simulink model "model_user_tracking"  (R2023a)
settings: Solver=VariableStepAuto  StartTime=0.0  StopTime=10.0  RelTol=1e-3
InitFcn:
  | f = 20%Hz
  | Robot_Start = [0,0];
  | User_Start = [-1,-1];
  | User_Speed = 1;
  | D_Accuracy = 0.25;
  | A_Accuracy = 10/180 * pi;
undefined symbols (not defined in the file or in its folder): DiscIntNeverNeededParam
libraries: dspsigops x2, eeGeneralControl x2
settings Model: Creator=Jordan  LastModifiedBy=Jordan

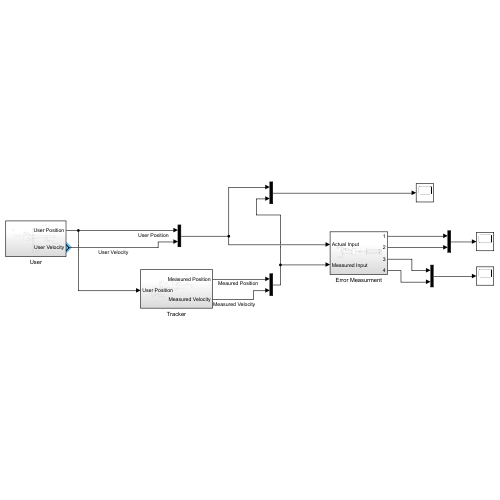
[thumbnail: Simulink's stored preview of the top-level diagram]
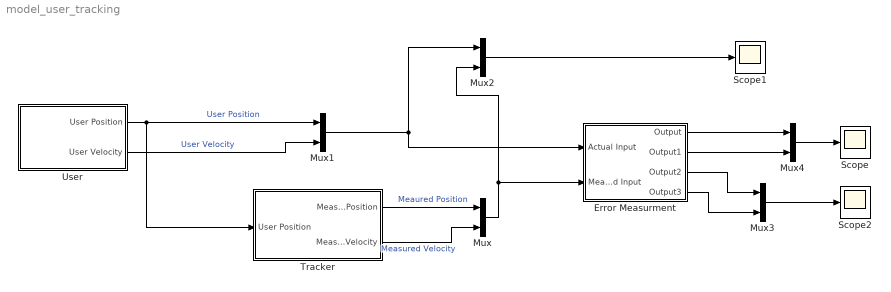
== system model_user_tracking ==
  Error Measurment : Subsystem
  Mux{,1..4} (5 alike) : Mux  Inputs=2
  Scope : Scope
  Scope1 : Scope
  Scope2 : Scope
  Tracker : Subsystem
  User : Subsystem
  wires:
  User/1(User Position) -> Mux1/1, Tracker/1(User Position)  "User Position"
  Tracker/2(Measured Velocity) -> Mux/2  "Measured Velocity"
  Tracker/1(Measured Position) -> Mux/1  "Meaured Position"
  User/2(User Velocity) -> Mux1/2  "User Velocity"
  Mux1/1 -> Mux2/1, Error Measurment/1("Actual Input ")
  Mux/1 -> Mux2/2, Error Measurment/2(Measured Input)
  Mux2/1 -> Scope1/1
  Error Measurment/1(Output) -> Mux4/1
  Error Measurment/2(Output1) -> Mux4/2
  Error Measurment/3(Output2) -> Mux3/1
  Error Measurment/4(Output3) -> Mux3/2
  Mux4/1 -> Scope/1
  Mux3/1 -> Scope2/1

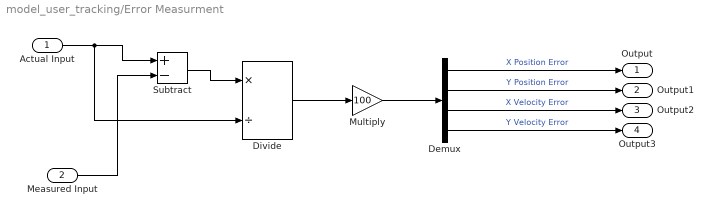
== system model_user_tracking/Error Measurment ==
  "Actual Input " : Inport
  Measured Input : Inport  Port=2
  Demux : Demux
  Divide : Product  Inputs=*/
  Multiply : Gain  Gain=100
  Subtract : Sum  Inputs=+-
  Output : Outport
  Output1 : Outport  Port=2
  Output2 : Outport  Port=3
  Output3 : Outport  Port=4
  wires:
  "Actual Input "/1 -> Divide/2, Subtract/1
  Measured Input/1 -> Subtract/2
  Subtract/1 -> Divide/1
  Divide/1 -> Multiply/1
  Multiply/1 -> Demux/1
  Demux/1 -> Output/1  "X Position Error"
  Demux/2 -> Output1/1  "Y Position Error"
  Demux/3 -> Output2/1  "X Velocity Error"
  Demux/4 -> Output3/1  "Y Velocity Error"

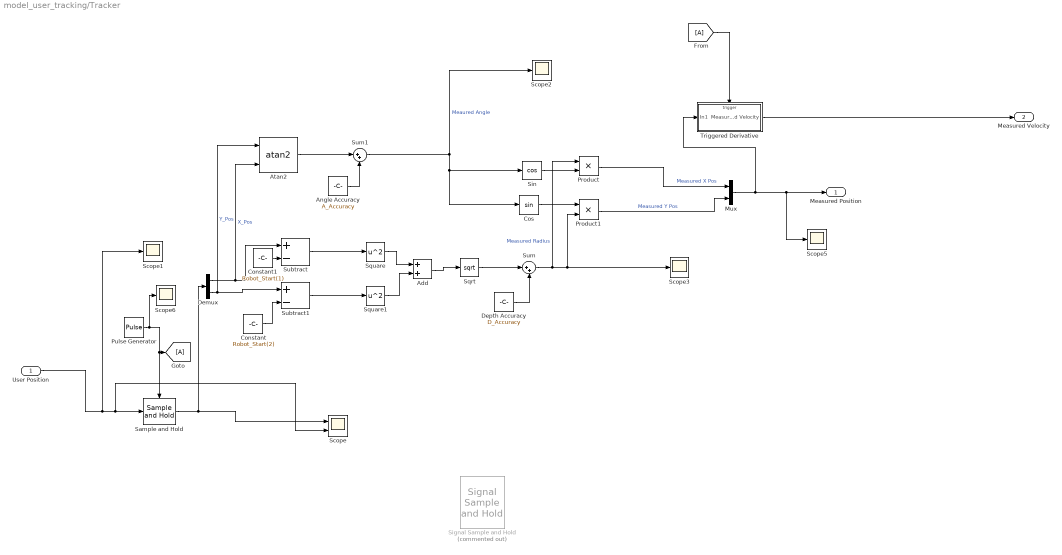
== system model_user_tracking/Tracker ==
  User Position : Inport
  Add : Sum
  Angle Accuracy : Constant  Value=A_Accuracy
  Atan2 : Trigonometry  Operator=atan2
  Constant : Constant  Value=Robot_Start(2)
  Constant1 : Constant  Value=Robot_Start(1)
  Cos : Trigonometry
  Demux : Demux  Outputs=2
  Depth Accuracy : Constant  Value=D_Accuracy
  From : From
  Goto : Goto
  Mux : Mux  Inputs=2
  Product : Product
  Product1 : Product
  Pulse Generator : DiscretePulseGenerator  PulseType=Time based  Period=1/f  PulseWidth=30
  Sample and Hold : dspsigops/Sample and Hold  trig=Rising edge  initCond=0  latchinput=off
  Scope : Scope  NumInputPorts=2
  Scope{1..3,5..6} (5 alike) : Scope
  Signal Sample and Hold : eeGeneralControl/Signal Sample and Hold  Commented=on  LabelModeActiveChoice=Discrete  x0=0  Ts=-1
      settings: LibrarySourceBlock=ee_sl_lib/General Control/Signal Sample and Hold
  Sin : Trigonometry  Operator=cos
  Sqrt : Sqrt
  Square : Math  Operator=square
  Square1 : Math  Operator=square
  Subtract : Sum  Inputs=+-
  Subtract1 : Sum  Inputs=+-
  Sum : Sum  Inputs=|++
  Sum1 : Sum  Inputs=|++
  Triggered Derivative : Subsystem
  Measured Position : Outport
  Measured Velocity : Outport  Port=2
  wires:
  User Position/1 -> Scope1/1, Sample and Hold/1, Scope/2
  Subtract1/1 -> Square1/1
  Subtract/1 -> Square/1
  Square/1 -> Add/1
  Square1/1 -> Add/2
  Add/1 -> Sqrt/1
  Demux/1 -> Atan2/2, Subtract/1  "X_Pos"
  Demux/2 -> Atan2/1, Subtract1/1  "Y_Pos"
  Constant/1 -> Subtract1/2
  Constant1/1 -> Subtract/2
  Sqrt/1 -> Sum/1
  Depth Accuracy/1 -> Sum/2
  Sum/1 -> Product/1, Product1/2, Scope3/1  "Measured Radius"
  Atan2/1 -> Sum1/1
  Angle Accuracy/1 -> Sum1/2
  Sum1/1 -> Cos/1, Sin/1, Scope2/1  "Meaured Angle"
  Sin/1 -> Product/2
  Cos/1 -> Product1/1
  Product1/1 -> Mux/2  "Measured Y Pos"
  Product/1 -> Mux/1  "Measured X Pos"
  Mux/1 -> Triggered Derivative/1(In1), Scope5/1, Measured Position/1
  From/1 -> Triggered Derivative/Trigger
  Sample and Hold/1 -> Demux/1, Scope/1
  Pulse Generator/1 -> Scope6/1, Goto/1, Sample and Hold/Trigger
  Triggered Derivative/1(Measured Velocity) -> Measured Velocity/1

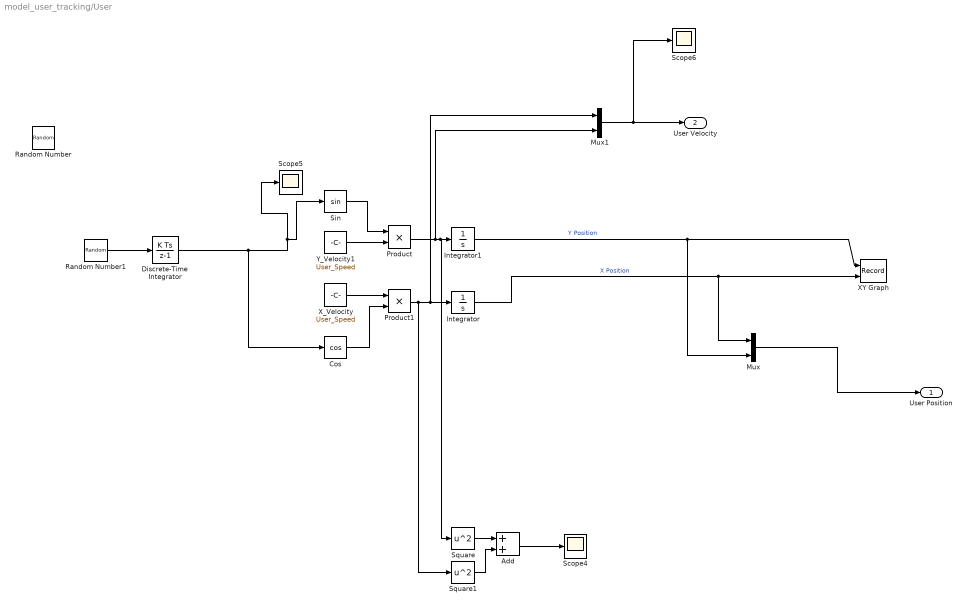
== system model_user_tracking/User ==
  Add : Sum
  Cos : Trigonometry  Operator=cos
  Discrete-Time Integrator : DiscreteIntegrator  SampleTime=0.25  ICPrevOutput=DiscIntNeverNeededParam  ICPrevScaledInput=DiscIntNeverNeededParam
  Integrator : Integrator  InitialCondition=User_Start(1)  LimitOutput=on  UpperSaturationLimit=3  LowerSaturationLimit=-3
  Integrator1 : Integrator  InitialCondition=User_Start(2)  LimitOutput=on  UpperSaturationLimit=3  LowerSaturationLimit=-3
  Mux : Mux  Inputs=2
  Mux1 : Mux  Inputs=2
  Product : Product
  Product1 : Product
  Random Number : RandomNumber  Variance=0.0378  Seed=123  SampleTime=0.25
  Random Number1 : RandomNumber  Variance=(pi)^2  Seed=123  SampleTime=0.2
  Scope4 : Scope
  Scope5 : Scope
  Scope6 : Scope
  Sin : Trigonometry
  Square : Math  Operator=square
  Square1 : Math  Operator=square
  XY Graph : Record  FileSettingsInternal="{\"entries\":[{\"content\":{\"excelSettings\":{\"content\":{},\"type\":\"Streamout.ExcelSettings\"}},\"type\":\"Streamout.FileSettingStorage\",\"uuid\":\"a6b072e3-8661-45ec-9a97-5f121e125176\"}],\"packageUris\":[\"http://schema.mathworks.com/mf0/streamout_blocks/R2020a\"],\"version\":\"1.0\"}"  Layout=[1 1]  SignalsInternal="{\"entries\":[{\"content\":{\"signals\":[{\"content\":{\"blockPath\":[\"model_user_tracking/User/XY Graph\"],\"dimensions\":[1],\"domain\":\"model_user_tracking/User/XY Graph\",\"lineColor\":\"#a2142f\",\"plots\":[1],\"port\":1,\"sid\":[\"\"],\"signalID\":899,\"signalName\":\"Y Position\"},\"type\":\"RecordBlkView.Signal\",\"uuid\":\"74513278-eac0-4257-8082-df148a71b635\"},{\"content\":{\"blockPath\":[\"model_user_tracking/User/XY Graph\"],\"dimensions\":[1],\"domain\":\"model_user_tracking/User/XY Graph\",\"lineColor\":\"#139fff\",\"plots\":[1],\"port\":2,\"sid\":[\"\"],\"signalID\":903,\"signalName\":\"X Position\"},\"type\":\"RecordBlkView.Signal\",\"uuid\":\"1db519f6-9f44-45c7-a46e-d80f2882f1bb\"}]},\"type\":\"RecordBlkView.InputSignals\",\"uuid\":\"e5429777-53db-4332-a7fb-7ba1e7e20543\"}],\"packageUris\":[\"http://schema.mathworks.com/mf0/streamout_blocks/R2020a\"],\"version\":\"1.0\"}"  VisualizationBindings="{\"xyplotplugin\":{\"info\":[{\"series\":[{\"bindingParametersList\":[{\"parameter\":\"X-Axis\",\"signalID\":899,\"signalName\":\"Y Position\"},{\"parameter\":\"Y-Axis\",\"signalID\":903,\"signalName\":\"X Position\"}],\"seriesID\":28698}],\"subplotID\":1}]}}"  CompatibilityTag=XY
  X_Velocity : Constant  Value=User_Speed
  Y_Velocity1 : Constant  Value=User_Speed
  User Position : Outport
  User Velocity : Outport  Port=2
  wires:
  Mux/1 -> User Position/1
  Y_Velocity1/1 -> Product/2
  Sin/1 -> Product/1
  X_Velocity/1 -> Product1/1
  Cos/1 -> Product1/2
  Product1/1 -> Square1/1, Mux1/1, Integrator/1
  Integrator1/1 -> Mux/2, XY Graph/1  "Y Position"
  Integrator/1 -> Mux/1, XY Graph/2  "X Position"
  Product/1 -> Mux1/2, Square/1, Integrator1/1
  Square/1 -> Add/1
  Square1/1 -> Add/2
  Add/1 -> Scope4/1
  Discrete-Time Integrator/1 -> Cos/1, Scope5/1, Sin/1
  Random Number1/1 -> Discrete-Time Integrator/1
  Mux1/1 -> Scope6/1, User Velocity/1

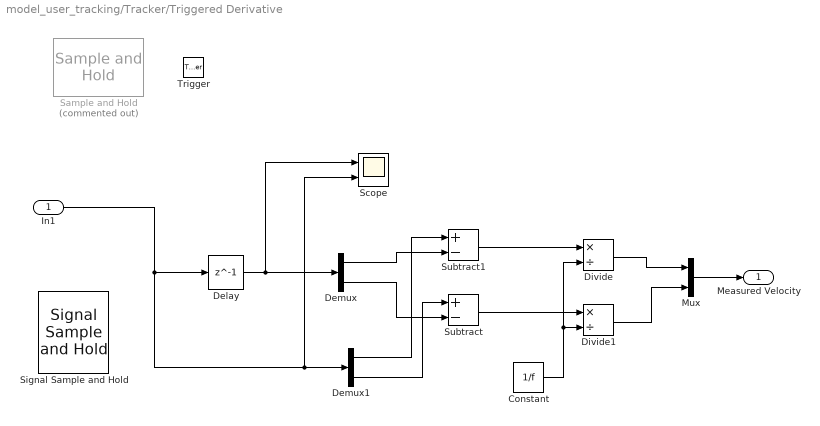
== system model_user_tracking/Tracker/Triggered Derivative ==
  In1 : Inport
  Trigger : TriggerPort  VariantControl=(inherit)  ShowOutputPort=on  OutputDataType=double  ZeroCross=off  InitialTriggerSignalState=zero  PortDimensions=1
  Constant : Constant  Value=1/f
  Delay : Delay  DelayLength=1
  Demux : Demux  Outputs=2
  Demux1 : Demux  Outputs=2
  Divide : Product  Inputs=*/
  Divide1 : Product  Inputs=*/
  Mux : Mux  Inputs=2
  Sample and Hold : dspsigops/Sample and Hold  Commented=on  trig=Rising edge  initCond=0  latchinput=on
  Scope : Scope  NumInputPorts=2
  Signal Sample and Hold : eeGeneralControl/Signal Sample and Hold  LabelModeActiveChoice=Discrete  x0=0  Ts=-1
      settings: LibrarySourceBlock=ee_sl_lib/General Control/Signal Sample and Hold
  Subtract : Sum  Inputs=+-
  Subtract1 : Sum  Inputs=+-
  Measured Velocity : Outport
  wires:
  Subtract1/1 -> Divide/1
  Subtract/1 -> Divide1/1
  Constant/1 -> Divide/2, Divide1/2
  Divide/1 -> Mux/1
  Divide1/1 -> Mux/2
  Mux/1 -> Measured Velocity/1
  In1/1 -> Scope/2, Demux1/1, Delay/1
  Delay/1 -> Scope/1, Demux/1
  Demux/2 -> Subtract/2
  Demux/1 -> Subtract1/2
  Demux1/1 -> Subtract1/1
  Demux1/2 -> Subtract/1
